simulink model "simulate_DSBTC"  (R2021a)
settings: Solver=VariableStepAuto  StartTime=0.0  StopTime=1  RelTol=1e-3
InitFcn:
  | fs = 4000;
  | frameSize = 512;
libraries: dspsrcs4 x2
settings Model: Creator=Byung-Jun Jang  LastModifiedBy=user
settings SolverCC: AlgebraicLoopSolver=TrustRegion
settings DataIOCC: ReturnWorkspaceOutputs=off
settings DebuggingCC: SFMachineParentedDataDiag=warning  ArithmeticOperatorsInVariantConditions=warning
settings SFSimCC: SimUseLocalCustomCode=off  CustomCodeUndefinedFunction=UseInterfaceOnly
settings RTWCC: RTWUseLocalCustomCode=off
settings CodeAppCC: StateflowObjectComments=on
settings SimscapeCC: SimscapeNormalizeSystem=off

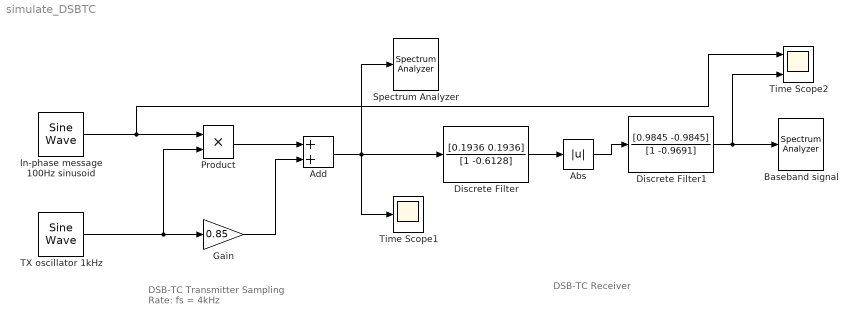
== system simulate_DSBTC ==
  note: DSB-TC Transmitter
      | Sampling Rate: fs = 4kHz
  note: DSB-TC Receiver
  Abs : Abs
  Add : Sum
  Baseband signal : SpectrumAnalyzer
  Discrete Filter : DiscreteFilter  Numerator=[0.1936 0.1936]  Denominator=[1 -0.6128]  InputProcessing=Columns as channels (frame based)  FilterStructure=Direct form II transposed  a0EqualsOne=on
  Discrete Filter1 : DiscreteFilter  Numerator=[0.9845 -0.9845]  Denominator=[1 -0.9691]  InputProcessing=Columns as channels (frame based)  FilterStructure=Direct form II transposed  a0EqualsOne=on
  Gain : Gain  Gain=0.85
  In-phase message 100Hz sinusoid : dspsrcs4/Sine Wave  Amplitude=1  Frequency=100  Phase=90  SampleMode=Discrete  OutComplex=Real  CompMethod=Trigonometric fcn  TableSize=Speed  SampleTime=1/fs  SamplesPerFrame=frameSize  ResetState=Restart at time zero  OutputFrames=off  dataType=double  wordLen=16  udDataType=sfix(16)  fracBitsMode=Best precision  numFracBits=15  OutDataTypeStr=double  LastOutDataTypeStr=double
  Product : Product
  Spectrum Analyzer : SpectrumAnalyzer
  TX oscillator 1kHz : dspsrcs4/Sine Wave  Amplitude=1  Frequency=1000  Phase=0  SampleMode=Discrete  OutComplex=Real  CompMethod=Trigonometric fcn  TableSize=Speed  SampleTime=1/fs  SamplesPerFrame=frameSize  ResetState=Restart at time zero  OutputFrames=off  dataType=double  wordLen=16  udDataType=sfix(16)  fracBitsMode=Best precision  numFracBits=15  OutDataTypeStr=double  LastOutDataTypeStr=double
  Time Scope1 : Scope
  Time Scope2 : Scope  NumInputPorts=2
  wires:
  In-phase message 100Hz sinusoid/1 -> Time Scope2/1, Product/1
  Add/1 -> Time Scope1/1, Spectrum Analyzer/1, Discrete Filter/1
  TX oscillator 1kHz/1 -> Product/2, Gain/1
  Abs/1 -> Discrete Filter1/1
  Product/1 -> Add/1
  Gain/1 -> Add/2
  Discrete Filter1/1 -> Time Scope2/2, Baseband signal/1
  Discrete Filter/1 -> Abs/1
